simulink model "LATC_Test_Calc"  (R2021b)
settings: Solver=FixedStepDiscrete  StartTime=3849.7586  StopTime=3889.7825  FixedStep=0.01  RelTol=1e-3
values from neighbouring files (symbols this model uses):
  P_Global_CharSpd_ms : value not decoded    [PubParsGlobal.sldd]
  P_Global_SteeringAngleRatio : value not decoded    [PubParsGlobal.sldd]
  P_Global_WheelBase_m : value not decoded    [PubParsGlobal.sldd]
  P_LCS_CycleTime = 0.4 0.4 0.4 0.4 0.4 0.4 0.4 0.4 0.4 0.6 0.6 0.6 0.6 0.6 0.6 0.6 0.4 0.4 0.4 0.4 0.4 0.4 0.4 0.4 0.4 0.6 0.6 0.6 0.6 0.6 0.6 0.6 0.4 0.4 0.4 0.4 0.4 0.4 0.4 0.4 0.4 0.6 0.6 0.6 0.6 0.6 0.6 0.6 0.4 0.4 0.4 0.4 0.4 0.4 0.4 0.4 0.4 0.6 0.6 0.6 0.6 0.6 0.6 0.6 0.4 0.4 0.4 0.4 0.4 0.4 0.4 0.4 0.4 0.6 0.6 0.6 0.6 0.6 0.6 0.6 0.4 0.4 0.4 0.4 0.4 0.4 0.4 0.4 0.4 0.6 0.6 0.6 0.6 0.6 0.6 0.6 0.4 0.4 0.4 0.4    [LATC.sldd]
  P_LCS_ESS_AngleSlope_Limit = 2.9    [LATC.sldd]    (also in LCS_v05.sldd)
  P_LCS_LATC_CurOffsetVehicleSpdLimitValue_degs = 7.0    [LATC.sldd]
  P_LCS_LATC_ELKAngleSlope_ratio : value not decoded    [LATC.sldd]
  P_LCS_LATC_ELKMaxLatAcc_ms2 : value not decoded    [LATC.sldd]
  P_LCS_LATC_ESSAngleSlope_ratio : value not decoded    [LATC.sldd]
  P_LCS_LATC_ESSMaxLatAcc_ms2 : value not decoded    [LATC.sldd]
  P_LCS_LATC_LCAngleSlope_ratio : value not decoded    [LATC.sldd]
  P_LCS_LATC_LCCancleMaxLatAcc_ms2 : value not decoded    [LATC.sldd]
  P_LCS_LATC_LCEcoAngleSlope_ratio : value not decoded    [LATC.sldd]
  P_LCS_LATC_LCEcoMaxLatAcc_ms2 : value not decoded    [LATC.sldd]
  P_LCS_LATC_LCKAngleSlope_ratio : value not decoded    [LATC.sldd]
  P_LCS_LATC_LCKIEAngleSlope_ratio : value not decoded    [LATC.sldd]
  P_LCS_LATC_LCKIEMaxLatAcc_ms2 : value not decoded    [LATC.sldd]
  P_LCS_LATC_LCKMaxLatAcc_ms2 : value not decoded    [LATC.sldd]
  P_LCS_LATC_LCNormalAngleSlope_ratio : value not decoded    [LATC.sldd]
  P_LCS_LATC_LCNormalMaxLatAcc_ms2 : value not decoded    [LATC.sldd]
  P_LCS_LATC_LCSportAngleSlope_ratio : value not decoded    [LATC.sldd]
  P_LCS_LATC_LCSportMaxLatAcc_ms2 : value not decoded    [LATC.sldd]
  P_LCS_LATC_LKAAngleSlope_ratio : value not decoded    [LATC.sldd]
  P_LCS_LATC_LKAMaxLatAcc_ms2 : value not decoded    [LATC.sldd]
  P_LCS_LATC_MatrixQ1_st = 0.8 0.8 1.2 1.4 1.4 1.4 2.0 2.2 2.2 2.2 2.2 2.2 2.2 2.2 2.2 2.2 0.8 0.8 1.2 1.4 1.4 1.4 2.0 2.2 2.2 2.2 2.2 2.2 2.2 2.2 2.2 2.2 0.8 0.8 1.2 1.4 1.4 1.4 2.0 2.2 2.2 2.2 2.2 2.2 2.2 2.2 2.2 2.2 0.8 0.8 1.2 1.4 1.4 1.4 2.0 2.2 2.2 2.2 2.2 2.2 2.2 2.2 2.2 2.2 0.8 0.8 1.2 1.4 1.4 1.4 2.0 2.2 2.2 2.2 2.2 2.2 2.2 2.2 2.2 2.2 0.8 0.8 1.2 1.4 1.4 1.4 2.0 2.2 2.2 2.2 2.2 2.2 2.2 2.2 2.2 2.2 0.8 0.8 1.2 1.4    [LATC.sldd]
  P_LCS_LATC_MatrixQ3_st = 20.0 20.0 20.0 20.0 20.0 15.0 15.0 15.0 15.0 15.0 15.0 15.0 15.0 13.0 13.0 13.0 20.0 20.0 20.0 20.0 20.0 15.0 15.0 15.0 15.0 15.0 15.0 15.0 15.0 13.0 13.0 13.0 20.0 20.0 20.0 20.0 20.0 15.0 15.0 15.0 15.0 15.0 15.0 15.0 15.0 13.0 13.0 13.0 20.0 20.0 20.0 20.0 20.0 15.0 15.0 15.0 15.0 15.0 15.0 15.0 15.0 13.0 13.0 13.0 20.0 20.0 20.0 20.0 20.0 15.0 15.0 15.0 15.0 15.0 15.0 15.0 15.0 13.0 13.0 13.0    [LATC.sldd]
  P_LCS_LATC_MatrixR_st = 10.0 10.0 10.0 10.0 10.0 10.0 10.0 15.0 15.0 15.0 15.0 15.0 15.0 15.0 15.0 15.0 10.0 10.0 10.0 10.0 10.0 10.0 10.0 15.0 15.0 15.0 15.0 15.0 15.0 15.0 15.0 15.0 10.0 10.0 10.0 10.0 10.0 10.0 10.0 15.0 15.0 15.0 15.0 15.0 15.0 15.0 15.0 15.0 10.0 10.0 10.0 10.0 10.0 10.0 10.0 15.0 15.0 15.0 15.0 15.0 15.0 15.0 15.0 15.0 10.0 10.0 10.0 10.0 10.0 10.0 10.0 15.0 15.0 15.0 15.0 15.0 15.0 15.0 15.0 15.0    [LATC.sldd]
  P_LCS_LATC_StateActivAngleSlopeLimit_ratio : value not decoded    [LATC.sldd]
  P_LCS_LATC_StateActiveFlg_TabX_st : value not decoded    [LATC.sldd]
  P_LCS_LATC_StateActiveHoldTime_TabY_st : value not decoded    [LATC.sldd]
  P_LCS_LATC_StateHoldTime_st = 250.0    [LATC.sldd]
  P_LCS_LATC_TarAngleFliterWindowSize = 5.0    [LATC.sldd]
  P_LCS_LineVaildSW = 0.0    [LATC.sldd]
  P_LCS_Lookahead_Distance : value not decoded    [LATC.sldd]
  P_LCS_VehicleSpd_TabX_Kph : value not decoded    [LATC.sldd]
libraries: simulink x4
(part 1 of 4)
settings Model: DataDictionary=LATC.sldd  Creator=GW00216231  LastModifiedBy=GW00216231
settings SolverCC: AlgebraicLoopSolver=TrustRegion
settings OptimizationCC: DefaultParameterBehavior=Inlined  EnhancedBackFolding=on  PassReuseOutputArgsThreshold=0  OptimizeBlockOrder=speed  DifferentSizesBufferReuse=on  OptimizationCustomize=off
settings DebuggingCC: SignalResolutionControl=TryResolveAllWithWarning  ParameterTunabilityLossMsg=error  SFMachineParentedDataDiag=warning  UnderSpecifiedDimensionMsg=warning
settings SFSimCC: MATLABDynamicMemAlloc=off
settings RTWCC: Description=Vector CANape/vSignalyzer Target (Visual C/C++ Project Makefile)  SystemTargetFile=cnp.tlc  TemplateMakefile=cnp_msdll.tmf
settings CodeAppCC: ForceParamTrailComments=on  OperatorAnnotations=on
settings STFCustomTargetCC: TargetLangStandard=C99 (ISO)  MATLABClassNameForMDSCustomization=Simulink.SoftwareTarget.TargetSpecificTriggerConfigurationBase  SystemTargetFile=cnp.tlc

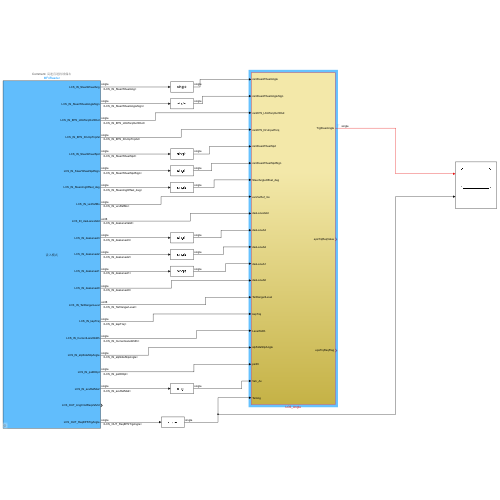
[thumbnail: Simulink's stored preview of the top-level diagram]
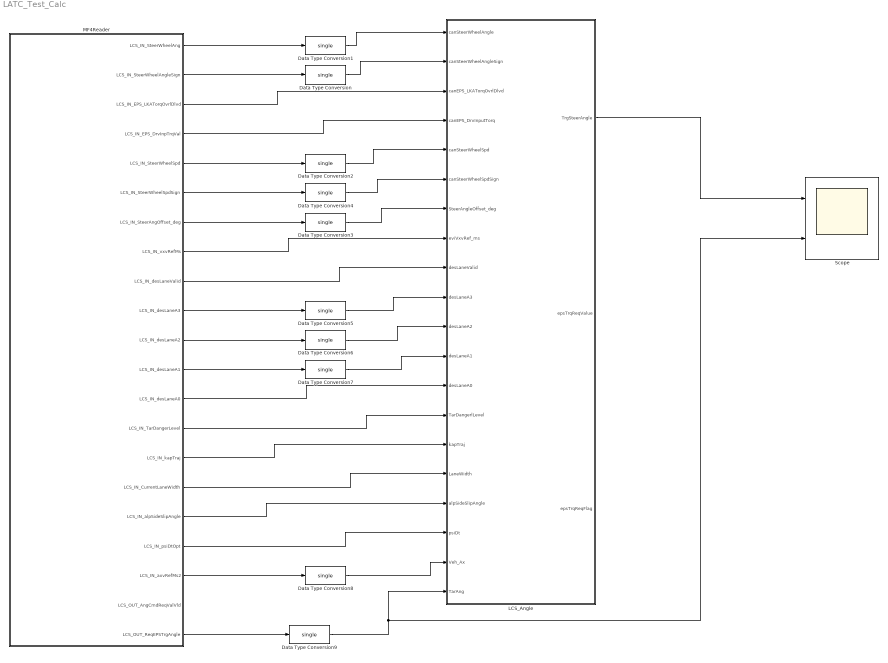
== system LATC_Test_Calc ==
  Data Type Conversion{,1..9} (10 alike) : DataTypeConversion  OutDataTypeStr=single
  LCS_Angle : Subsystem
  MF4Reader : Subsystem  Description=Comment: 高速直道持续偏右  mask(MF4Reader(Bata1.5)){pfileName=F:\04_APE_Temple_Files\ADAS_CAN+dll+SimulinkModel\TrajectoryPoints_Track_Test2\Data_Recorder\NOH_IDC_V71_0049_2021-12-31-16-17-22.mf4, LoadFilter={'Checksum','RollingCounter','AEB','HAVP_','^P_','BSW','Reserved','PACK','autosar','LM_','exec','fid_stat','g_swc','_PIL_','_TLJ_','_PP_','SPID','DMON','gen_init','JAPedObj','^MAC','CAN_DataFrame','DIAG','CAL'}, CaseSensitive=off, AutoDataTypeConvert=off, FunMod=读入模式, SearchSeed=[], BackGroundColorRead=lightBlue, BackGroundColorPort=white, StopTime=3889.7825, StartTime=3849.7586}
      mask prompts: pfileName "mf4文件:"; LoadFilter "加载过滤:"; CaseSensitive "搜索大小写敏感"; AutoDataTypeConvert "自动数据类型转换"; FunMod "模式选择"; SearchSeed "搜索："; StopTime "数据结束时间"; StartTime "数据开始时间"
      mask help: 该模块可将选择的mdf文件中包含的信号以列表形式读取出来，读入模式下，该模块将用户选择的信号读取成matlab时间序列，并导入simulink用于仿真。接口模式下，该模块将以用户选择的信号名添加CANape仿真用接口，用于dll生成（需要安装CANape simulink addon）。点击"帮助"了解更多。
      settings: AttributesFormatString=%<Description>
      mask Help:
      | Version：Bata1.5  Date: 20211012 Editor: Chengzhenning
      | 当前为测试版，可能存在不稳定或性能问题，建议/Bug反馈请联系Editor，谢谢。
      | 
      | 使用简述：
      | Step1:检查加载过滤。(若如特殊需求无需设置此项)
      | Step2:选取MF4文件
      | Setp3:点击Load/Refresh，加载mf4数据中的信号
      | Step4:选取信号（操作同bus selector，支持搜索）
      | Step5:选择模式及是否自动添加数据类型转换
      | Step6:点击Add添加接口
      | 
      | 数据导入：
      | 选择文件：支持mdf mf4文件，支持中文路径
      | 加载过滤：加载过滤是将符合过滤条件(标准matlab正则表达式)的所有信号跳过，过滤后在“全部信号”中无法找到，可配置多个过滤条件，多个条件以元胞数组的形式输入，例如{'表达式1'，'表达式2'} ，可根据情况自行修改。不建议删除默认的加载过滤条件。
      | 
      | 自定义设置项说明：
      | 读入模式：当配置为导入mdf数据后，该模块会将已选择的信号从mdf文件中读取出来，存入base workspace。并在模型中使用fromworkspace调用。
      | 接口模式：当配置为生成ape接口时，将按照已选择的信号名生成ape仿真用接口模块。
      | 自动数据类型转换：设置为自动数据类型转换之后将在内部自动添加data type conversion，请务必规定后端使用的数据类型，否者以读出或输入的数据类型直出。
      | 
      | 搜索：
      | 搜索：搜索支持常用通配符（同ape），当搜索条件为空或点击输入框的取消后将重置搜索结果，搜索条件请在弹出的输入框中输入；
      | 
      | 其他提醒：
      | 因版本限制，自定义设置部分请用右侧按钮进行设置，左侧仅作显示用；
      | 因版本限制，搜索条件请在弹出的输入框中输入；
      | 加载数据后，该模块会自动将仿真起止时间设置为所有有效数据的最大起止时间区间，仿真步长需要自行设置；
      | 
      | 故障解决：
      | 若发生接口混乱的情况，点击不常用设置->ClearPorts！删除所有模块后重新添加。
      | 若存在其他报错问题，尝试执行clear all（所有工作区将被清除，注意保存数据！！！）后重新load数据。
      | 若提醒找不到变，在没有clear all的前提下，重新Add即可。若执行了clear all，需要点击Load重新加载数据。
      | 
      | 兼容性：
      | 兼容20b和21a，但因2020b兼容性问题，部分参数只能使用对话框的形式输入而不能直接修改，Matlab 21a版本体验更佳。若需要21a版，请联系Editor。
      | 
      | 警告：
      | 删除默认的加载过滤条件可能会导致错误，不建议删除默认的加载过滤条件！
      | 每个模型中只能同时使用一个MF4Reader !
      | 尽量不要手动清空工作区，clear之后需求重新add，clear all之后需要重新load并add
      | 
      | 更新记录：
      | 1 Bata1.0  Date 20210927 Editor Chengzhenning
      |    初版发布
      | 2 Bata1.1  Date 20210929 Editor Chengzhenning
      |    优化个别无法读取的信号的检测过滤,提高对数据的兼容性，bug反馈人：温俊亮
      | 3 Bata1.2  Date 20210930 Editor Chengzhenning
      |    修复重调整接口会导致外部连线混乱的问题，不再使用弹窗提醒找不到的信号，bug反馈人：王亚伟
      | 4.Bata1.3  Date 20210930 Editor Chengzhenning
      |    自动添加信号名，提升加载数据速度
      | 5.Bata1.4  Date 20211009 Editor Chengzhenning
      |    增加内部的自动信号类型转换，可配置。支持设置搜索是否大小写敏感。更改设置工作模式的位置，不必每次都设置。
      | 6.Bata1.5  Date 20211012 Editor Chengzhenning
      |    适配2021b，不再兼容2020b以下。其他操作逻辑优化，更易使用。
      | 
      | 感谢所有提供bug反馈和功能建议的用户！
      mask TypeOptions FunMod: 读入模式 | 接口模式
      mask DialogControl ParameterGroupVar Prompt: 数据源选择
      mask DialogControl Control2 Prompt: 选择文件
      mask DialogControl Control2 Callback:
      | global fileobj;
      | 
      | [Name,directory] = uigetfile('*.mf4;*.mdf','Choose a mf4-file');
      | if isequal(Name,0) || isequal(directory,0)
      |     disp('User pressed cancel')
      |     return;
      | else
      |     fName=fullfile(directory,Name);
      |     if strcmp(fName,get_param(gcb,'pfileName'))&&~isempty(fileobj)
      |         return;
      |     end
      |     set_param(gcb,'pfileName',fName);
      |     disp(['User selected ',fName ])
      | end
      | 
      | 
      | commentStr=NaN;
      | StartTime=0;
      | StopTime=30;
      | if ~isempty(Simulink.Mask.get(gcb).Parameters(2).Value)
      |     LoadExclude=eval(Simulink.Mask.get(gcb).Parameters(2).Value);
      |     if ~iscell(LoadExclude)
      |         msgbox('加载过滤必须是元胞字符串数组或空值！');
      |         return;
      |     end
      | else
      |     LoadExclude={};
      | end
      | fName=Simulink.Mask.get(gcb).Parameters(1).Value;
      | if ~exist(fName)
      |     msgbox('文件不存在！');
      |     return;
      | end
      | t1=clock;
      | disp('-----------------------------');
      | disp(['打开文件:',fName,'中...']);
      | bar = waitbar(0,'正在读取数据...0%');
      | fileobj=mdf(fName);
      | disp(['打开完成，用时',num2str(etime(clock,t1)),'秒']);
      | %commentStr=native2unicode(unicode2native(fileobj.Comment,'windows-1252'));%20b以下版本用
      | commentStr=fileobj.Comment;
      | disp(['数据备注:',commentStr]);
      | t1=clock;
      | disp('读取信号中...');
      | ALLSigNames={};
      | ALLSigsGroup={};
      | ChannelNamesNum=length(fileobj.ChannelNames);
      | timeflag=true;
      | for i=2:ChannelNamesNum
      |     if ishandle(bar)
      |         str=['正在加载数据...',num2str(fix(100*i/ChannelNamesNum)),'%'];
      |         waitbar(i/ChannelNamesNum,bar,str,'Interpreter','none');
      |     end
      |     if fileobj.ChannelGroup(i).DataSize==0
      |         continue;
      |     end
      |     for m=1:length(fileobj.ChannelNames{i})
      |         ChannelName=fileobj.ChannelNames{i}{m};
      |         if (ChannelName=='t')
      |             continue;
      |         end
      |         if isempty(ChannelName)
      |             continue;
      |         end
      |         ExcludeFlag=false;
      |         for x=1:length(LoadExclude)
      |             if regexp(ChannelName,LoadExclude{x})
      |                 ExcludeFlag=true;
      |             end
      |         end
      |         if ExcludeFlag
      |             continue;
      |         end
      |         try
      |             temp=read(fileobj,i,ChannelName,'OutputFormat','Timeseries');
      |         catch
      |             disp([ChannelName,'不支持读入,已跳过！']);
      |         end
      |         if isempty(temp)
      |             continue;
      |         end
      |         timelength=temp.TimeInfo.end-temp.TimeInfo.start;
      |         if timelength<=0
      |             continue;
      |         end
      |         if timeflag
      |             StartTime=temp.TimeInfo.start;
      |             StopTime=temp.TimeInfo.end;
      |             timeflag=false;
      |         else
      |             if StartTime>temp.TimeInfo.start
      |                 StartTime=temp.TimeInfo.start;
      |             end
      |             if StopTime<temp.TimeInfo.end
      |                 StopTime=temp.TimeInfo.end;
      |             end
      |         end
      | 
      |         ALLSigNames=[ALLSigNames,ChannelName];
      |         ALLSigsGroup=[ALLSigsGroup,num2str(i)];
      |     end
      | end
      | 
      | %set_param(gcs,'StartTime',num2str(StartTime));
      | %set_param(gcs,'StopTime',num2str(StopTime));
      | set_param(gcb,'StartTime',num2str(StartTime));
      | set_param(gcb,'StopTime',num2str(StopTime));
      | waitbar(1,bar,['加载结束，信号数量：',num2str(length(ALLSigNames))],'Interpreter','none');
      | pause(2);
      | if ishandle(bar)
      |     close(bar);
      | end
      | if isempty(ALLSigNames)
      |     msgbox('读取数据失败！');
      |     disp('异常结束!');
      |     return;
      | else
      |     %commentStr=native2unicode(unicode2native(fileobj.Comment,'windows-1252'));
      |     disp(['读取完成,','信号数量：',num2str(length(ALLSigNames)),',用时',num2str(etime(clock,t1)),'秒']);
      |     disp(['数据起止时间为[',num2str(StartTime),' , ',num2str(StopTime),']']);
      |     disp('Finish!');
      | end
      | disp('-----------------------------');
      | set_param(gcb,'Description',['Comment: ',commentStr]);
      | 
      | 
      | maskObj = Simulink.Mask.get( gcb );
      | ControlALLSigsGroup= maskObj.getDialogControl('ALLSigsGroup');
      | ControlALLSigNames= maskObj.getDialogControl('ALLSigNames');
      | treeControlL = maskObj.getDialogControl('Control3');
      | treeControlR = maskObj.getDialogControl('Control6');
      | 
      | ControlALLSigsGroup.TreeItems=ALLSigsGroup;
      | ControlALLSigNames.TreeItems=ALLSigNames;
      | treeControlL.TreeItems=ALLSigNames;
      | 
      | selAllSig=treeControlR.TreeItems();
      | if isempty(selAllSig)
      |     return;
      | end
      | for i= 1:length(selAllSig)
      |     if max(strfind(selAllSig{i},'???'))>0
      |         if ismember(selAllSig{i}(4:end),ALLSigNames)
      |             selAllSig{i}=selAllSig{i}(4:end);
      |         end
      |     else
      |         if ~ismember(selAllSig{i},ALLSigNames)
      |             selAllSig{i}=['???',selAllSig{i}];
      |         end
      |     end
      | end
      | treeControlR.TreeItems=selAllSig;
      mask DialogControl Container11 Prompt: 自定义设置
      mask DialogControl SearchButton Prompt: Search
      mask DialogControl SearchButton Callback:
      | maskObj = Simulink.Mask.get( gcb );
      | treeControlL = maskObj.getDialogControl('Control3');
      | ControlALLSigNames= maskObj.getDialogControl('ALLSigNames');
      | ALLSigNames=ControlALLSigNames.TreeItems();
      | 
      | SearchSeed= get_param(gcb,'SearchSeed');
      | SearchSeed=strrep(SearchSeed,'[','');
      | SearchSeed=strrep(SearchSeed,']','');
      | SLsiglist={};
      | if isempty(SearchSeed)
      |     treeControlL.TreeItems=ALLSigNames;
      |     return;
      | end
      | CaseSensitive=get_param(gcb,'CaseSensitive');
      | if CaseSensitive=="off"
      |     for i=1:length(ALLSigNames)
      |         if regexpi(ALLSigNames{i},regexptranslate('wildcard',SearchSeed))
      |             %if regexp(ALLSigNames{i},SerchSeed)
      |             SLsiglist=[SLsiglist,ALLSigNames{i}];
      |         end
      |     end
      | else
      |     for i=1:length(ALLSigNames)
      |         if regexp(ALLSigNames{i},regexptranslate('wildcard',SearchSeed))
      |         %   if regexp(ALLSigNames{i},SerchSeed)
      |             SLsiglist=[SLsiglist,ALLSigNames{i}];
      |         end
      |     end
      | end
      | treeControlL.TreeItems=SLsiglist;
      mask DialogControl Control3 Prompt: 所有信号
      mask DialogControl Control9 Prompt: Load
      mask DialogControl Control9 Callback:
      | global fileobj;
      | 
      | commentStr=NaN;
      | StartTime=0;
      | StopTime=30;
      | if ~isempty(Simulink.Mask.get(gcb).Parameters(2).Value)
      |     LoadExclude=eval(Simulink.Mask.get(gcb).Parameters(2).Value);
      |     if ~iscell(LoadExclude)
      |         msgbox('加载过滤必须是元胞字符串数组或空值！');
      |         return;
      |     end
      | else
      |     LoadExclude={};
      | end
      | fName=Simulink.Mask.get(gcb).Parameters(1).Value;
      | if ~exist(fName)
      |     msgbox('文件不存在！');
      |     return;
      | end
      | t1=clock;
      | disp('-----------------------------');
      | disp(['打开文件:',fName,'中...']);
      | bar = waitbar(0,'正在读取数据...0%');
      | fileobj=mdf(fName);
      | disp(['打开完成，用时',num2str(etime(clock,t1)),'秒']);
      | %commentStr=native2unicode(unicode2native(fileobj.Comment,'windows-1252'));%20b以下版本用
      | commentStr=fileobj.Comment;
      | disp(['数据备注:',commentStr]);
      | t1=clock;
      | disp('读取信号中...');
      | ALLSigNames={};
      | ALLSigsGroup={};
      | ChannelNamesNum=length(fileobj.ChannelNames);
      | timeflag=true;
      | for i=2:ChannelNamesNum
      |     if ishandle(bar)
      |         str=['正在加载数据...',num2str(fix(100*i/ChannelNamesNum)),'%'];
      |         waitbar(i/ChannelNamesNum,bar,str,'Interpreter','none');
      |     end
      |     if fileobj.ChannelGroup(i).DataSize==0
      |         continue;
      |     end
      |     for m=1:length(fileobj.ChannelNames{i})
      |         ChannelName=fileobj.ChannelNames{i}{m};
      |         if (ChannelName=='t')
      |             continue;
      |         end
      |         if isempty(ChannelName)
      |             continue;
      |         end
      |         ExcludeFlag=false;
      |         for x=1:length(LoadExclude)
      |             if regexp(ChannelName,LoadExclude{x})
      |                 ExcludeFlag=true;
      |             end
      |         end
      |         if ExcludeFlag
      |             continue;
      |         end
      |         try
      |             temp=read(fileobj,i,ChannelName,'OutputFormat','Timeseries');
      |         catch
      |             disp([ChannelName,'不支持读入,已跳过！']);
      |         end
      |         if isempty(temp)
      |             continue;
      |         end
      |         timelength=temp.TimeInfo.end-temp.TimeInfo.start;
      |         if timelength<=0
      |             continue;
      |         end
      |         if timeflag
      |             StartTime=temp.TimeInfo.start;
      |             StopTime=temp.TimeInfo.end;
      |             timeflag=false;
      |         else
      |             if StartTime>temp.TimeInfo.start
      |                 StartTime=temp.TimeInfo.start;
      |             end
      |             if StopTime<temp.TimeInfo.end
      |                 StopTime=temp.TimeInfo.end;
      |             end
      |         end
      | 
      |         ALLSigNames=[ALLSigNames,ChannelName];
      |         ALLSigsGroup=[ALLSigsGroup,num2str(i)];
      |     end
      | end
      | 
      | %set_param(gcs,'StartTime',num2str(StartTime));
      | %set_param(gcs,'StopTime',num2str(StopTime));
      | set_param(gcb,'StartTime',num2str(StartTime));
      | set_param(gcb,'StopTime',num2str(StopTime));
      | waitbar(1,bar,['加载结束，信号数量：',num2str(length(ALLSigNames))],'Interpreter','none');
      | pause(2);
      | if ishandle(bar)
      |     close(bar);
      | end
      | if isempty(ALLSigNames)
      |     msgbox('读取数据失败！');
      |     disp('异常结束!');
      |     return;
      | else
      |     %commentStr=native2unicode(unicode2native(fileobj.Comment,'windows-1252'));
      |     disp(['读取完成,','信号数量：',num2str(length(ALLSigNames)),',用时',num2str(etime(clock,t1)),'秒']);
      |     disp(['数据起止时间为[',num2str(StartTime),' , ',num2str(StopTime),']']);
      |     disp('Finish!');
      | end
      | disp('-----------------------------');
      | set_param(gcb,'Description',['Comment: ',commentStr]);
      | 
      | 
      | maskObj = Simulink.Mask.get( gcb );
      | ControlALLSigsGroup= maskObj.getDialogControl('ALLSigsGroup');
      | ControlALLSigNames= maskObj.getDialogControl('ALLSigNames');
      | treeControlL = maskObj.getDialogControl('Control3');
      | treeControlR = maskObj.getDialogControl('Control6');
      | 
      | ControlALLSigsGroup.TreeItems=ALLSigsGroup;
      | ControlALLSigNames.TreeItems=ALLSigNames;
      | treeControlL.TreeItems=ALLSigNames;
      | 
      | selAllSig=treeControlR.TreeItems();
      | if isempty(selAllSig)
      |     return;
      | end
      | for i= 1:length(selAllSig)
      |     if max(strfind(selAllSig{i},'???'))>0
      |         if ismember(selAllSig{i}(4:end),ALLSigNames)
      |             selAllSig{i}=selAllSig{i}(4:end);
      |         end
      |     else
      |         if ~ismember(selAllSig{i},ALLSigNames)
      |             selAllSig{i}=['???',selAllSig{i}];
      |         end
      |     end
      | end
      | treeControlR.TreeItems=selAllSig;
      mask DialogControl Control7 Prompt: Select >>
      mask DialogControl Control7 Callback:
      | maskObj = Simulink.Mask.get( gcb );
      | treeControlL = maskObj.getDialogControl('Control3');
      | treeControlR = maskObj.getDialogControl('Control6');
      | 
      | seld=treeControlL.getSelectedItems();
      | if isempty(seld)
      |     return;
      | end
      | if ismember(seld,treeControlR.TreeItems)
      |     msgbox('信号重复')
      | end
      | treeControlR.TreeItems=unique([treeControlR.TreeItems,seld'],'stable');
      | treeControlR.setSelectedItems(seld);
      mask DialogControl Control6 Prompt: 已选信号
      mask DialogControl up Prompt: Up
      mask DialogControl up Callback:
      | maskObj = Simulink.Mask.get(gcb);
      | treeControlR = maskObj.getDialogControl('Control6');
      | RSig=treeControlR.TreeItems();
      | SelectSig=treeControlR.getSelectedItems();
      | 
      | if isempty(SelectSig)
      |     return;
      | end
      | 
      | [~,selIndex]=ismember(SelectSig,RSig);
      | 
      | if min(selIndex)>2
      |     AllSigPart3=RSig(1:min(selIndex)-2);
      | else
      |     AllSigPart3={};
      | end
      | RSig(selIndex)=[];
      | [~,Part1Index]=ismember(AllSigPart3,RSig);
      | RSig(Part1Index)=[];
      | 
      | treeControlR.TreeItems=[AllSigPart3,SelectSig',RSig];
      | treeControlR.setSelectedItems(SelectSig);
      mask DialogControl down Prompt: Down
      mask DialogControl down Callback:
      | maskObj = Simulink.Mask.get(gcb);
      | treeControlR = maskObj.getDialogControl('Control6');
      | RSig=treeControlR.TreeItems();
      | SelectSig=treeControlR.getSelectedItems();
      | 
      | if isempty(SelectSig)
      |     return;
      | end
      | 
      | [~,selIndex]=ismember(SelectSig,RSig);
      | 
      | if max(selIndex)+2<=length(RSig)
      |     AllSigPart3=RSig(max(selIndex)+2:end);
      | else
      |     AllSigPart3={};
      | end
      | RSig(selIndex)=[];
      | [~,Part3Index]=ismember(AllSigPart3,RSig);
      | RSig(Part3Index)=[];
      | 
      | treeControlR.TreeItems=[RSig,SelectSig',AllSigPart3];
      | treeControlR.setSelectedItems(SelectSig);
      mask DialogControl Control11 Prompt: Remove
      mask DialogControl Control11 Callback:
      | maskObj = Simulink.Mask.get(gcb);
      | treeControlR = maskObj.getDialogControl('Control6');
      | AllSig=treeControlR.TreeItems();
      | SelectSig=treeControlR.getSelectedItems();
      | if ~isempty(SelectSig)
      |     [~,DelIndex]=ismember(SelectSig,AllSig);
      |     AllSig(DelIndex)=[];
      | end
      | treeControlR.TreeItems=AllSig;
      mask DialogControl Control8 Prompt: Add
      mask DialogControl Control8 Callback:
      | global fileobj
      | if isempty(fileobj)
      |     msgbox('数据丢失，请重新load！');
      |     return;
      | end
      | FunMod=get_param(gcb,'FunMod');
      | %检查是否存在未识别到的信号
      | maskObj = Simulink.Mask.get( gcb );
      | treeControlL = maskObj.getDialogControl('Control3');
      | treeControlR = maskObj.getDialogControl('Control6');
      | ControlALLSigsGroup= maskObj.getDialogControl('ALLSigsGroup');
      | ControlALLSigNames= maskObj.getDialogControl('ALLSigNames');
      | ControlOldSigName= maskObj.getDialogControl('OldSigName');
      | 
      | DataSelect=treeControlR.TreeItems();
      | ALLSigsGroup=ControlALLSigsGroup.TreeItems();
      | ALLSigNames=ControlALLSigNames.TreeItems();
      | OldSigName=ControlOldSigName.TreeItems();
      | 
      | if isempty(DataSelect)
      |     msgbox('未选择信号！');
      |     return;
      | end
      | if isempty(DataSelect)
      |     return;
      | end
      | if ~iscell(ALLSigNames)
      |     ALLSigNames={};
      | end
      | for i= 1:length(DataSelect)
      |     if max(strfind(DataSelect{i},'???'))>0
      |         if ismember(DataSelect{i}(4:end),ALLSigNames)
      |             DataSelect{i}=DataSelect{i}(4:end);
      |         end
      |     else
      |         if ~ismember(DataSelect{i},ALLSigNames)
      |             DataSelect{i}=['???',DataSelect{i}];
      |         end
      |     end
      | end
      | treeControlR.TreeItems=DataSelect;
      | signotfind=false;
      | for i= 1:length(DataSelect)
      |     if max(strfind(DataSelect{i},'???'))>0
      |         signotfind=true;
      |     end
      | end
      | if signotfind
      |     signotfindresp=questdlg('存在已选的信号无法找到！请刷新数据或检查数据中是否存在这些信号','错误提醒','跳过无法找到的信号','停止添加接口','停止添加接口');
      |     if isempty(signotfindresp) || signotfindresp == "停止添加接口"
      |         return;
      |     end
      | end
      | 
      | oldPos=get_param(gcb,'Position');%记忆位置，防止游走
      | %定义模块路径方便使用
      | FunctionBlockPath = 'simulink/User-Defined Functions/Interpreted MATLAB Function';
      | OutPortBlockPath ='simulink/Commonly Used Blocks/Out1';
      | SaturationPath ='simulink/Discontinuities/Saturation';
      | ConstantPath = 'simulink/Sources/Constant';
      | DIPath = 'simulink/Discrete/Discrete-Time Integrator';
      | FromWorkSpacePath = 'simulink/Sources/From Workspace';
      | CANapeInputPath='canapelib/CANape I//O/Input';
      | DataTypeConversionPath='simulink/Signal Attributes/Data Type Conversion';
      | 
      | %添加模块前先删除所有模块和连线
      | set_param(gcb,'BackGroundColor','white');
      | SourceList=find_system(gcb,'LookUnderMasks','on','SearchDepth',1,'BlockType','FromWorkspace');
      | if ~isempty(SourceList)
      |     for i=1:length(SourceList)
      |         delete_block(SourceList{i});
      |     end
      | end
      | LinesList=find_system(gcb,'LookUnderMasks','on','FindAll','on','type','line');
      | if ~isempty(LinesList)
      |     for i=1:length(LinesList)
      |         if ishandle(LinesList(i))
      |             delete_line(LinesList(i));
      |         end
      |     end
      | end
      | 
      | SysList=find_system(gcb,'LookUnderMasks','on','SearchDepth',1,'BlockType','SubSystem');
      | if length(SysList)>1
      |     for i=2:length(SysList)
      |         delete_block(SysList{i});
      |     end
      | end
      | DataTypeConversionsList=find_system(gcb,'LookUnderMasks','on','SearchDepth',1,'BlockType','DataTypeConversion');
      | if ~isempty(DataTypeConversionsList)
      |     for i=1:length(DataTypeConversionsList)
      |         delete_block(DataTypeConversionsList{i});
      |     end
      | end
      | %添加信号源
      | SourceBlockSum=0;
      | added_block={};
      | if ~isempty(OldSigName)
      |     for i=1:length(OldSigName);
      |         evalin('base',['clear ',OldSigName{i}]);
      |     end
      | end
      | AutoDataTypeConvert=get_param(gcb,'AutoDataTypeConvert');
      | 
      | if FunMod=="读入模式" %fromworkspace
      |     for j=1:length(DataSelect)
      |         SigName=DataSelect{j};
      |         temp=strrep(SigName,'.','_');
      |         temp=strrep(temp,'[','_');
      |         temp=strrep(temp,']','_');
      |         if length(temp)>60
      |             temp=temp(length(temp)-59:end);
      |         end
      |         SigAliasName=['s_',temp];
      |         [SigExist,Sigindex]= ismember(SigName,ALLSigNames);
      |         if SigExist
      |             sigGroupIndex=str2double(ALLSigsGroup{Sigindex});
      |         else
      |             disp(['未找到信号: ',SigName,' ，已跳过！']);
      |             continue;
      |         end
      |         %添加模块
      |         Swidth=100;
      |         Shigh=30;
      |         Owidth=30;
      |         Ohigh=14;
      |         Sdy=30;
      |         SOdx=800;
      |         SDdx=250;
      |         temp=read(fileobj,sigGroupIndex,SigName,'OutputFormat','Timeseries');
      |         assignin('base',SigAliasName,temp);
      |         Source=add_block(FromWorkSpacePath,[gcb,'/' ,'sourceValue_',SigName],'Interpolate','off','VariableName',SigAliasName,'OutputAfterFinalValue','Setting to zero', ...
      |             'Position',[0,(Shigh)*SourceBlockSum+SourceBlockSum*Sdy, Swidth ,(Shigh)*(SourceBlockSum+1)+SourceBlockSum*Sdy]);
      |         if AutoDataTypeConvert=="on"
      |             DataTypeConversion=add_block(DataTypeConversionPath,[gcb,'/' ,'Convert_',SigName], ...
      |                 'Position',[SDdx,(Shigh)*SourceBlockSum+SourceBlockSum*Sdy, SDdx+Swidth ,(Shigh)*(SourceBlockSum+1)+SourceBlockSum*Sdy]);
      |         end
      |         Out=find_system(gcb,'LookUnderMasks','on','SearchDepth',1,'BlockType','Outport','PortName',SigName);
      |         if isempty(Out)
      |             Out=add_block(OutPortBlockPath,[gcb,'/' ,SigName],...
      |                 'Position',[SOdx,0.5*(Shigh-Ohigh)+(Ohigh)*SourceBlockSum+SourceBlockSum*(Sdy+Shigh-Ohigh),SOdx+Owidth ,0.5*(Shigh-Ohigh)+(Ohigh)*(SourceBlockSum+1)+SourceBlockSum*(Sdy+Shigh-Ohigh)]);
      |         else
      |             Out=Out{1};
      |             set_param(Out,'Port',num2str(SourceBlockSum+1),'Position',[SOdx,0.5*(Shigh-Ohigh)+(Ohigh)*SourceBlockSum+SourceBlockSum*(Sdy+Shigh-Ohigh),SOdx+Owidth ,0.5*(Shigh-Ohigh)+(Ohigh)*(SourceBlockSum+1)+SourceBlockSum*(Sdy+Shigh-Ohigh)]);
      |         end
      |         if AutoDataTypeConvert=="on"
      |             add_line(gcb,get_param(Source,'PortHandles').Outport,get_param(DataTypeConversion,'PortHandles').Inport)
      |             line=add_line(gcb,get_param(DataTypeConversion,'PortHandles').Outport,get_param(Out,'PortHandles').Inport);
      |         else
      |             line=add_line(gcb,get_param(Source,'PortHandles').Outport,get_param(Out,'PortHandles').Inport);
      |         end
      |         set_param(line,'Name',SigName);
      |         SourceBlockSum=SourceBlockSum+1;
      |         set_param(get_param(gcb,'PortHandles').Outport(SourceBlockSum),'ShowPropagatedSignals','on');
      |         OldSigName{j}=SigAliasName;
      |     end
      |     set_param(gcb,'BackGroundColor',get_param(gcb,'BackGroundColorRead'));
      |     set_param(gcs,'StartTime',get_param(gcb,'StartTime'));
      |     set_param(gcs,'StopTime',get_param(gcb,'StopTime'));
      |     disp('读入数据完成，已经自动设置模型仿真时间为数据起止时间');
      | elseif FunMod=="接口模式"
      |     for j=1:length(DataSelect)
      |         SigName=DataSelect{j};
      |         temp=strrep(SigName,'.','_');
      |         if length(temp)>60
      |             temp=temp(length(temp)-59:end);
      |         end
      |         SigAliasName=['s_',temp];
      |         [SigExist,Sigindex]= ismember(SigName,ALLSigNames);
      |         if SigExist
      |             sigGroupIndex=ALLSigsGroup{Sigindex};
      |         else
      |             disp(['未找到信号: ',SigName,' ，已跳过！']);
      |             continue
      |         end
      |         %添加模块
      |         Swidth=100;
      |         Shigh=30;
      |         Owidth=30;
      |         Ohigh=14;
      |         Sdy=30;
      |         SOdx=800;
      |         SDdx=250;
      |         try
      |         Source=add_block('canapelib/CANape I//O/Input',[gcb,'/' ,'sourceValue_',SigName],...
      |             'envName',SigName,'Position',[0,(Shigh)*SourceBlockSum+SourceBlockSum*Sdy, Swidth ,(Shigh)*(SourceBlockSum+1)+SourceBlockSum*Sdy]);
      |         catch
      |             msgbox('可能未安装CANape Simulink Add-on！无法添加接口，已终止！')
      |             return;
      |         end
      |         if AutoDataTypeConvert=="on"
      |             DataTypeConversion=add_block(DataTypeConversionPath,[gcb,'/' ,'Convert_',SigName], ...
      |                 'Position',[SDdx,(Shigh)*SourceBlockSum+SourceBlockSum*Sdy-10, SDdx+Swidth ,(Shigh)*(SourceBlockSum+1)+SourceBlockSum*Sdy-10]);
      |         end
      |         Out=find_system(gcb,'LookUnderMasks','on','SearchDepth',1,'BlockType','Outport','PortName',SigName);
      |         if isempty(Out)
      |             Out=add_block(OutPortBlockPath,[gcb,'/' ,SigName],...
      |                 'Position',[SOdx,0.5*(Shigh-Ohigh)+(Ohigh)*SourceBlockSum+SourceBlockSum*(Sdy+Shigh-Ohigh)-10,SOdx+Owidth ,0.5*(Shigh-Ohigh)+(Ohigh)*(SourceBlockSum+1)+SourceBlockSum*(Sdy+Shigh-Ohigh)-10]);
      |         else
      |             Out=Out{1};
      |             set_param(Out,'Port',num2str(SourceBlockSum+1),'Position',[SOdx,0.5*(Shigh-Ohigh)+(Ohigh)*SourceBlockSum+SourceBlockSum*(Sdy+Shigh-Ohigh)-10,SOdx+Owidth ,0.5*(Shigh-Ohigh)+(Ohigh)*(SourceBlockSum+1)+SourceBlockSum*(Sdy+Shigh-Ohigh)-10]);
      |         end
      |         if AutoDataTypeConvert=="on"
      |             add_line(gcb,get_param(Source,'PortHandles').Outport(1),get_param(DataTypeConversion,'PortHandles').Inport)
      |             line=add_line(gcb,get_param(DataTypeConversion,'PortHandles').Outport,get_param(Out,'PortHandles').Inport);
      |         else
      |             line=add_line(gcb,get_param(Source,'PortHandles').Outport(1),get_param(Out,'PortHandles').Inport);
      |         end
      |         set_param(line,'Name',SigName);
      |         SourceBlockSum=SourceBlockSum+1;
      |         set_param(get_param(gcb,'PortHandles').Outport(SourceBlockSum),'ShowPropagatedSignals','on');
      |         OldSigName{j}=SigAliasName;
      |     end
      |     set_param(gcb,'BackGroundColor',get_param(gcb,'BackGroundColorPort'));
      |     set_param(gcs,'StartTime','0');
      |     disp('添加CANape接口完成，已经自动设置模型仿真开始时间为0');
      | end
      | ControlOldSigName.TreeItems=OldSigName;
      | % 删除多余output
      | OutList=find_system(gcb,'LookUnderMasks','on','SearchDepth',1,'BlockType','Outport');
      | if ~isempty(OutList)
      |     for i=1:length(OutList)
      |         if str2double(get_param(OutList{i},'Port'))>SourceBlockSum
      |             delete_block(OutList{i});
      |         end
      |     end
      | end
      | 
      | if (oldPos(4)-oldPos(2))/SourceBlockSum<20
      |     oldPos(4)=oldPos(2)+(SourceBlockSum+1)*20;
      | end
      | set_param(gcb,'Position',oldPos);
      mask DialogControl ccc Prompt: 其他不常用设置
      mask DialogControl Control17 Prompt: 记忆当前模式模块颜色
      mask DialogControl Control17 Callback:
      | FunMod=get_param(gcb,'FunMod');
      | if FunMod=="读入模式"
      |     set_param(gcb,'BackGroundColorRead',get_param(gcb,'BackGroundColor'));
      | end
      | if FunMod=="接口模式"
      |     set_param(gcb,'BackGroundColorPort',get_param(gcb,'BackGroundColor'));
      | end
      mask DialogControl Control25 Prompt: ClearPorts!
      mask DialogControl Control25 Callback:
      | SourceList=find_system(gcb,'LookUnderMasks','on','SearchDepth',1,'BlockType','FromWorkspace');
      | if ~isempty(SourceList)
      |     for i=1:length(SourceList)
      |         delete_block(SourceList{i});
      |     end
      | end
      | LinesList=find_system(gcb,'LookUnderMasks','on','FindAll','on','type','line');
      | if ~isempty(LinesList)
      |     for i=1:length(LinesList)
      |         if ishandle(LinesList(i))
      |             delete_line(LinesList(i));
      |         end
      |     end
      | end
      | 
      | SysList=find_system(gcb,'LookUnderMasks','on','SearchDepth',1,'BlockType','SubSystem');
      | if length(SysList)>1
      |     for i=2:length(SysList)
      |         delete_block(SysList{i});
      |     end
      | end
      | DataTypeConversionsList=find_system(gcb,'LookUnderMasks','on','SearchDepth',1,'BlockType','DataTypeConversion');
      | if ~isempty(DataTypeConversionsList)
      |     for i=1:length(DataTypeConversionsList)
      |         delete_block(DataTypeConversionsList{i});
      |     end
      | end
      | OutList=find_system(gcb,'LookUnderMasks','on','SearchDepth',1,'BlockType','Outport');
      | if ~isempty(OutList)
      |     for i=1:length(OutList)
      |         delete_block(OutList{i});
      |     end
      | end
      mask DialogControl Container13 Prompt: Debug
      mask DialogControl OldSigName Prompt: OldSigName
      mask DialogControl ALLSigNames Prompt: ALLSigNames
      mask DialogControl ALLSigsGroup Prompt: ALLSigsGroup
      mask Display:
      | FunMod=get_param(gcb,'FunMod');
      | SourceList=find_system(gcb,'LookUnderMasks','on','SearchDepth',1,'BlockType','FromWorkspace');
      | SysList=find_system(gcb,'LookUnderMasks','on','SearchDepth',1,'BlockType','SubSystem');
      | if ~isempty(SourceList)
      | disp('读入模式');
      | elseif length(SysList)>1
      |     disp('接口模式');
      | else
      |     disp('未添加接口');
      | end
  Scope : Scope  NumInputPorts=2
  wires:
  MF4Reader/1(LCS_IN_SteerWheelAng) -> Data Type Conversion1/1
  MF4Reader/2(LCS_IN_SteerWheelAngleSign) -> Data Type Conversion/1
  MF4Reader/3(LCS_IN_EPS_LKATorqOvrlDlvd) -> LCS_Angle/3(canEPS_LKATorqOvrlDlvd)
  MF4Reader/4(LCS_IN_EPS_DrvInpTrqVal) -> LCS_Angle/4(canEPS_DrvInputTorq)
  MF4Reader/5(LCS_IN_SteerWheelSpd) -> Data Type Conversion2/1
  MF4Reader/6(LCS_IN_SteerWheelSpdSign) -> Data Type Conversion4/1
  MF4Reader/7(LCS_IN_SteerAngOffset_deg) -> Data Type Conversion3/1
  MF4Reader/8(LCS_IN_vxvRefMs) -> LCS_Angle/8(eviVxvRef_ms)
  MF4Reader/9(LCS_IN_desLaneValid) -> LCS_Angle/9(desLaneValid)
  MF4Reader/10(LCS_IN_desLaneA3) -> Data Type Conversion5/1
  MF4Reader/11(LCS_IN_desLaneA2) -> Data Type Conversion6/1
  MF4Reader/12(LCS_IN_desLaneA1) -> Data Type Conversion7/1
  MF4Reader/13(LCS_IN_desLaneA0) -> LCS_Angle/13(desLaneA0)
  MF4Reader/14(LCS_IN_TarDangerLevel) -> LCS_Angle/14(TarDangerlLevel)
  MF4Reader/15(LCS_IN_kapTraj) -> LCS_Angle/15(kapTraj)
  MF4Reader/16(LCS_IN_CurrentLaneWidth) -> LCS_Angle/16(LaneWidth)
  MF4Reader/17(LCS_IN_alpSideSlipAngle) -> LCS_Angle/17(alpSideSlipAngle)
  MF4Reader/18(LCS_IN_psiDtOpt) -> LCS_Angle/18(psiDt)
  MF4Reader/19(LCS_IN_axvRefMs2) -> Data Type Conversion8/1
  Data Type Conversion1/1 -> LCS_Angle/1(canSteerWheelAngle)
  Data Type Conversion/1 -> LCS_Angle/2(canSteerWheelAngleSign)
  Data Type Conversion2/1 -> LCS_Angle/5(canSteerWheelSpd)
  Data Type Conversion3/1 -> LCS_Angle/7(SteerAngleOffset_deg)
  Data Type Conversion4/1 -> LCS_Angle/6(canSteerWheelSpdSign)
  Data Type Conversion7/1 -> LCS_Angle/12(desLaneA1)
  Data Type Conversion6/1 -> LCS_Angle/11(desLaneA2)
  Data Type Conversion5/1 -> LCS_Angle/10(desLaneA3)
  Data Type Conversion8/1 -> LCS_Angle/19(Veh_Ax)
  MF4Reader/21(LCS_OUT_ReqEPSTrgAngle) -> Data Type Conversion9/1
  Data Type Conversion9/1 -> Scope/2, LCS_Angle/20(TarAng)
  LCS_Angle/1(TrgSteerAngle) -> Scope/1

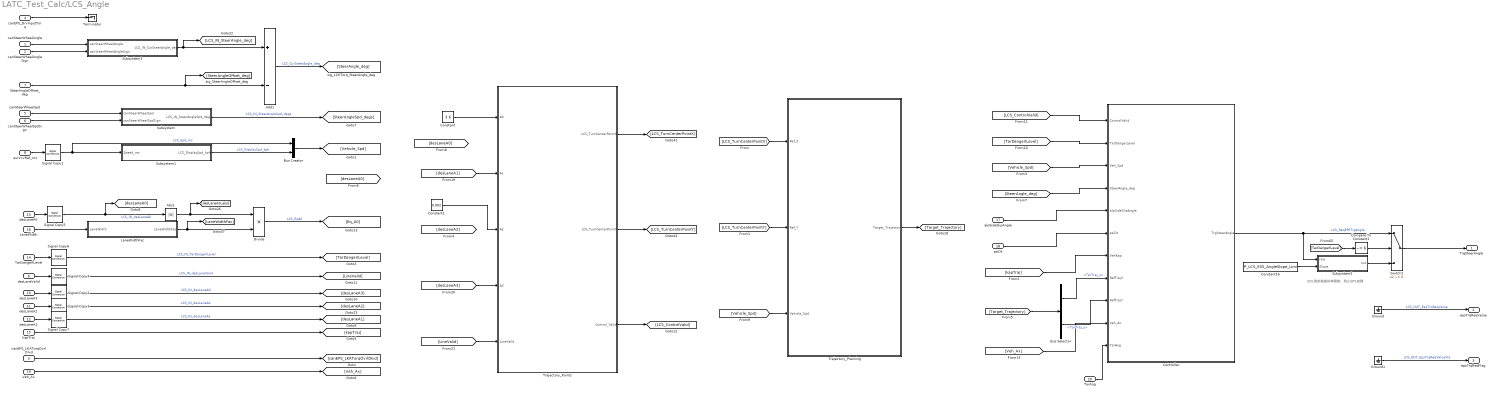
== system LATC_Test_Calc/LCS_Angle ==
  note: ESS请求角度斜率限制，防止EPS故障
  canSteerWheelAngle : Inport
  canSteerWheelAngleSign : Inport  Port=2
  canEPS_LKATorqOvrlDlvd : Inport  Port=3
  canEPS_DrvInputTorq : Inport  Port=4
  canSteerWheelSpd : Inport  Port=5
  canSteerWheelSpdSign : Inport  Port=6
  SteerAngleOffset_deg : Inport  Port=7
  eviVxvRef_ms : Inport  Port=8
  desLaneValid : Inport  Port=9
  desLaneA3 : Inport  Port=10
  desLaneA2 : Inport  Port=11
  desLaneA1 : Inport  Port=12
  desLaneA0 : Inport  Port=13
  TarDangerlLevel : Inport  Port=14
  kapTraj : Inport  Port=15
  LaneWidth : Inport  Port=16
  alpSideSlipAngle : Inport  Port=17
  psiDt : Inport  Port=18
  Veh_Ax : Inport  Port=19
  TarAng : Inport  Port=20
  Abs1 : Abs
  Add1 : Sum  Inputs=+-
  Bus Creator : BusCreator  Inputs=2
  Bus Selector : BusSelector  OutputSignals=TarTraj_x,TarTraj_y
  Compare To Constant1 : simulink/Logic and Bit Operations/Compare To Constant  relop=~=  const=6  OutDataTypeStr=boolean
  Constant : Constant  Value=3.6  OutDataTypeStr=single
  Constant1 : Constant  Value=0.002  OutDataTypeStr=single
  Constant16 : Constant  Description=2.9  Value=P_LCS_ESS_AngleSlope_Limit  OutDataTypeStr=single
      settings: AttributesFormatString=%<Description>
  Controller : Subsystem
  Divide : Product  Inputs=**
  Ground : Ground
  Ground1 : Ground
  LaneWidthFac : Subsystem
  Signal Copy{1..7} (7 alike) : SignalConversion  OverrideOpt=off
  Subsystem : Subsystem
  Subsystem1 : Subsystem
  Subsystem3 : Subsystem
  Subsystem5 : Subsystem
  Switch1 : Switch  Criteria=u2 ~= 0
  Terminator : Terminator
  Trajectory_Planning : Subsystem
  Trajectory_Points : Subsystem
  TrgSteerAngle : Outport  OutDataTypeStr=single
  epsTrqReqValue : Outport  Port=2
  epsTrqReqFlag : Outport  Port=3
  wires:
  Signal Copy4/1 -> [LineValid]  "LCS_IN_desLaneValid"
  canEPS_DrvInputTorq/1 -> Terminator/1
  desLaneA2/1 -> Signal Copy3/1
  Signal Copy5/1 -> Abs1/1, [desLaneA0]  "LCS_IN_desLaneA0"
  eviVxvRef_ms/1 -> Signal Copy1/1
  Add1/1 -> [SteerAngle_deg]  "LCS_CurSteerAngle_deg"
  canEPS_LKATorqOvrlDlvd/1 -> [canEPS_LKATorqOvrlDlvd]
  SteerAngleOffset_deg/1 -> Add1/2, [SteerAngleOffset_deg]
  kapTraj/1 -> [kapTraj]
  Abs1/1 -> Divide/1, [desLaneA0_abs]
  TarDangerlLevel/1 -> Signal Copy6/1
  Divide/1 -> [Eq_A0]  "LCS_EqA0"
  desLaneA0/1 -> Signal Copy5/1
  desLaneValid/1 -> Signal Copy4/1
  [TarDangerlLevel] -> Compare To Constant1/1
  Compare To Constant1/1 -> Switch1/2
  Switch1/1 -> TrgSteerAngle/1
  Subsystem5/1(out) -> Switch1/3
  Constant16/1 -> Subsystem5/2(Slope)
  Signal Copy6/1 -> [TarDangerlLevel]  "LCS_IN_TarDangerlLevel"
  Controller/1(TrgSteerAngle) -> Switch1/1, Subsystem5/1(raw)  "LCS_ReqEPSTrgAngle"
  Ground1/1 -> epsTrqReqFlag/1  "LCS_OUT_EpsTrqReqValueVld"
  Ground/1 -> epsTrqReqValue/1  "LCS_OUT_EpsTrqReqValue"
  [desLaneA1] -> Trajectory_Points/2(A1)
  [desLaneA3] -> Trajectory_Points/4(A3)
  [LineValid] -> Trajectory_Points/5(LineVaild)
  Trajectory_Points/1(LCS_TurnCenterPointX) -> [LCS_TurnCenterPointX]
  Trajectory_Points/2(LCS_TurnCenterPointY) -> [LCS_TurnCenterPointY]
  Trajectory_Points/3(Control_Valid) -> [LCS_ControlValid]
  LaneWidth/1 -> LaneWidthFac/1(LaneWidth)
  LaneWidthFac/1(LaneWidthFac) -> [LaneWidthFac], Divide/2
  canSteerWheelSpd/1 -> Subsystem/1(canSteerWheelSpd)
  canSteerWheelSpdSign/1 -> Subsystem/2(canSteerWheelSpdSign)
  Subsystem/1(LCS_IN_SteerAngleSpd_degs) -> [SteerAngleSpd_degs]  "LCS_IN_SteerAngleSpd_degs"
  Subsystem1/1(LCS_DisplaySpd_kph) -> Bus Creator/2  "LCS_DisplaySpd_kph"
  Subsystem3/1(LCS_IN_CurSteerAngle_deg) -> Add1/1, [LCS_IN_SteerAngle_deg]
  canSteerWheelAngle/1 -> Subsystem3/1(canSteerWheelAngle)
  canSteerWheelAngleSign/1 -> Subsystem3/2(canSteerWheelAngleSign)
  Signal Copy1/1 -> Bus Creator/1, Subsystem1/1(Speed_ms)  "LCS_Spd_ms"
  Bus Creator/1 -> [Vehicle_Spd]
  desLaneA3/1 -> Signal Copy2/1
  Signal Copy2/1 -> [desLaneA3]  "LCS_IN_desLaneA3"
  desLaneA1/1 -> Signal Copy7/1
  Signal Copy3/1 -> [desLaneA2]  "LCS_IN_desLaneA2"
  Signal Copy7/1 -> [desLaneA1]  "LCS_IN_desLaneA1"
  [LCS_TurnCenterPointX] -> Trajectory_Planning/1(Ref_X)
  [LCS_TurnCenterPointY] -> Trajectory_Planning/2(Ref_Y)
  [Vehicle_Spd] -> Trajectory_Planning/3(Vehicle_Spd)
  Trajectory_Planning/1(Target_Trajectory) -> [Target_Trajectory]
  [kapTraj] -> Controller/7(VehKap)
  [Vehicle_Spd] -> Controller/3(Veh_Spd)
  psiDt/1 -> Controller/6(psiDt)
  alpSideSlipAngle/1 -> Controller/5(alpSideSlipAngle)
  [Target_Trajectory] -> Bus Selector/1
  Bus Selector/1 -> Controller/8(RefTrajX)  "<TarTraj_x>"
  Bus Selector/2 -> Controller/9(RefTrajY)  "<TarTraj_y>"
  [SteerAngle_deg] -> Controller/4(SteerAngle_deg)
  [TarDangerlLevel] -> Controller/2(TarDangerLevel)
  [LCS_ControlValid] -> Controller/1(ControlValid)
  Veh_Ax/1 -> [Veh_Ax]
  [Veh_Ax] -> Controller/10(Veh_Ax)
  TarAng/1 -> Controller/11(TarAng)
  Constant1/1 -> Trajectory_Points/3(A2)
  Constant/1 -> Trajectory_Points/1(A0)

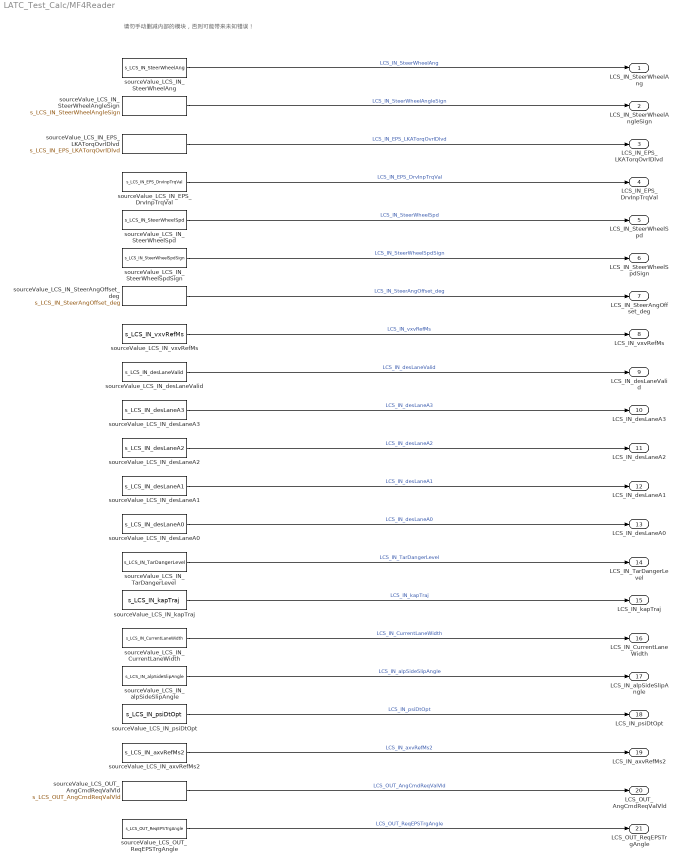
== system LATC_Test_Calc/MF4Reader ==
  note: 请勿手动删减内部的模块，否则可能带来未知错误！
  sourceValue_LCS_IN_CurrentLaneWidth : FromWorkspace  VariableName=s_LCS_IN_CurrentLaneWidth  Interpolate=off  OutputAfterFinalValue=Setting to zero
  sourceValue_LCS_IN_EPS_DrvInpTrqVal : FromWorkspace  VariableName=s_LCS_IN_EPS_DrvInpTrqVal  Interpolate=off  OutputAfterFinalValue=Setting to zero
  sourceValue_LCS_IN_EPS_LKATorqOvrlDlvd : FromWorkspace  VariableName=s_LCS_IN_EPS_LKATorqOvrlDlvd  Interpolate=off  OutputAfterFinalValue=Setting to zero
  sourceValue_LCS_IN_SteerAngOffset_deg : FromWorkspace  VariableName=s_LCS_IN_SteerAngOffset_deg  Interpolate=off  OutputAfterFinalValue=Setting to zero
  sourceValue_LCS_IN_SteerWheelAng : FromWorkspace  VariableName=s_LCS_IN_SteerWheelAng  Interpolate=off  OutputAfterFinalValue=Setting to zero
  sourceValue_LCS_IN_SteerWheelAngleSign : FromWorkspace  VariableName=s_LCS_IN_SteerWheelAngleSign  Interpolate=off  OutputAfterFinalValue=Setting to zero
  sourceValue_LCS_IN_SteerWheelSpd : FromWorkspace  VariableName=s_LCS_IN_SteerWheelSpd  Interpolate=off  OutputAfterFinalValue=Setting to zero
  sourceValue_LCS_IN_SteerWheelSpdSign : FromWorkspace  VariableName=s_LCS_IN_SteerWheelSpdSign  Interpolate=off  OutputAfterFinalValue=Setting to zero
  sourceValue_LCS_IN_TarDangerLevel : FromWorkspace  VariableName=s_LCS_IN_TarDangerLevel  Interpolate=off  OutputAfterFinalValue=Setting to zero
  sourceValue_LCS_IN_alpSideSlipAngle : FromWorkspace  VariableName=s_LCS_IN_alpSideSlipAngle  Interpolate=off  OutputAfterFinalValue=Setting to zero
  sourceValue_LCS_IN_axvRefMs2 : FromWorkspace  VariableName=s_LCS_IN_axvRefMs2  Interpolate=off  OutputAfterFinalValue=Setting to zero
  sourceValue_LCS_IN_desLaneA0 : FromWorkspace  VariableName=s_LCS_IN_desLaneA0  Interpolate=off  OutputAfterFinalValue=Setting to zero
  sourceValue_LCS_IN_desLaneA1 : FromWorkspace  VariableName=s_LCS_IN_desLaneA1  Interpolate=off  OutputAfterFinalValue=Setting to zero
  sourceValue_LCS_IN_desLaneA2 : FromWorkspace  VariableName=s_LCS_IN_desLaneA2  Interpolate=off  OutputAfterFinalValue=Setting to zero
  sourceValue_LCS_IN_desLaneA3 : FromWorkspace  VariableName=s_LCS_IN_desLaneA3  Interpolate=off  OutputAfterFinalValue=Setting to zero
  sourceValue_LCS_IN_desLaneValid : FromWorkspace  VariableName=s_LCS_IN_desLaneValid  Interpolate=off  OutputAfterFinalValue=Setting to zero
  sourceValue_LCS_IN_kapTraj : FromWorkspace  VariableName=s_LCS_IN_kapTraj  Interpolate=off  OutputAfterFinalValue=Setting to zero
  sourceValue_LCS_IN_psiDtOpt : FromWorkspace  VariableName=s_LCS_IN_psiDtOpt  Interpolate=off  OutputAfterFinalValue=Setting to zero
  sourceValue_LCS_IN_vxvRefMs : FromWorkspace  VariableName=s_LCS_IN_vxvRefMs  Interpolate=off  OutputAfterFinalValue=Setting to zero
  sourceValue_LCS_OUT_AngCmdReqValVld : FromWorkspace  VariableName=s_LCS_OUT_AngCmdReqValVld  Interpolate=off  OutputAfterFinalValue=Setting to zero
  sourceValue_LCS_OUT_ReqEPSTrgAngle : FromWorkspace  VariableName=s_LCS_OUT_ReqEPSTrgAngle  Interpolate=off  OutputAfterFinalValue=Setting to zero
  LCS_IN_SteerWheelAng : Outport
  LCS_IN_SteerWheelAngleSign : Outport  Port=2
  LCS_IN_EPS_LKATorqOvrlDlvd : Outport  Port=3
  LCS_IN_EPS_DrvInpTrqVal : Outport  Port=4
  LCS_IN_SteerWheelSpd : Outport  Port=5
  LCS_IN_SteerWheelSpdSign : Outport  Port=6
  LCS_IN_SteerAngOffset_deg : Outport  Port=7
  LCS_IN_vxvRefMs : Outport  Port=8
  LCS_IN_desLaneValid : Outport  Port=9
  LCS_IN_desLaneA3 : Outport  Port=10
  LCS_IN_desLaneA2 : Outport  Port=11
  LCS_IN_desLaneA1 : Outport  Port=12
  LCS_IN_desLaneA0 : Outport  Port=13
  LCS_IN_TarDangerLevel : Outport  Port=14
  LCS_IN_kapTraj : Outport  Port=15
  LCS_IN_CurrentLaneWidth : Outport  Port=16
  LCS_IN_alpSideSlipAngle : Outport  Port=17
  LCS_IN_psiDtOpt : Outport  Port=18
  LCS_IN_axvRefMs2 : Outport  Port=19
  LCS_OUT_AngCmdReqValVld : Outport  Port=20
  LCS_OUT_ReqEPSTrgAngle : Outport  Port=21
  wires:
  sourceValue_LCS_IN_SteerWheelAng/1 -> LCS_IN_SteerWheelAng/1  "LCS_IN_SteerWheelAng"
  sourceValue_LCS_IN_SteerWheelAngleSign/1 -> LCS_IN_SteerWheelAngleSign/1  "LCS_IN_SteerWheelAngleSign"
  sourceValue_LCS_IN_EPS_LKATorqOvrlDlvd/1 -> LCS_IN_EPS_LKATorqOvrlDlvd/1  "LCS_IN_EPS_LKATorqOvrlDlvd"
  sourceValue_LCS_IN_EPS_DrvInpTrqVal/1 -> LCS_IN_EPS_DrvInpTrqVal/1  "LCS_IN_EPS_DrvInpTrqVal"
  sourceValue_LCS_IN_SteerWheelSpd/1 -> LCS_IN_SteerWheelSpd/1  "LCS_IN_SteerWheelSpd"
  sourceValue_LCS_IN_SteerWheelSpdSign/1 -> LCS_IN_SteerWheelSpdSign/1  "LCS_IN_SteerWheelSpdSign"
  sourceValue_LCS_IN_SteerAngOffset_deg/1 -> LCS_IN_SteerAngOffset_deg/1  "LCS_IN_SteerAngOffset_deg"
  sourceValue_LCS_IN_vxvRefMs/1 -> LCS_IN_vxvRefMs/1  "LCS_IN_vxvRefMs"
  sourceValue_LCS_IN_desLaneValid/1 -> LCS_IN_desLaneValid/1  "LCS_IN_desLaneValid"
  sourceValue_LCS_IN_desLaneA3/1 -> LCS_IN_desLaneA3/1  "LCS_IN_desLaneA3"
  sourceValue_LCS_IN_desLaneA2/1 -> LCS_IN_desLaneA2/1  "LCS_IN_desLaneA2"
  sourceValue_LCS_IN_desLaneA1/1 -> LCS_IN_desLaneA1/1  "LCS_IN_desLaneA1"
  sourceValue_LCS_IN_desLaneA0/1 -> LCS_IN_desLaneA0/1  "LCS_IN_desLaneA0"
  sourceValue_LCS_IN_TarDangerLevel/1 -> LCS_IN_TarDangerLevel/1  "LCS_IN_TarDangerLevel"
  sourceValue_LCS_IN_kapTraj/1 -> LCS_IN_kapTraj/1  "LCS_IN_kapTraj"
  sourceValue_LCS_IN_CurrentLaneWidth/1 -> LCS_IN_CurrentLaneWidth/1  "LCS_IN_CurrentLaneWidth"
  sourceValue_LCS_IN_alpSideSlipAngle/1 -> LCS_IN_alpSideSlipAngle/1  "LCS_IN_alpSideSlipAngle"
  sourceValue_LCS_IN_psiDtOpt/1 -> LCS_IN_psiDtOpt/1  "LCS_IN_psiDtOpt"
  sourceValue_LCS_IN_axvRefMs2/1 -> LCS_IN_axvRefMs2/1  "LCS_IN_axvRefMs2"
  sourceValue_LCS_OUT_AngCmdReqValVld/1 -> LCS_OUT_AngCmdReqValVld/1  "LCS_OUT_AngCmdReqValVld"
  sourceValue_LCS_OUT_ReqEPSTrgAngle/1 -> LCS_OUT_ReqEPSTrgAngle/1  "LCS_OUT_ReqEPSTrgAngle"
